simulink model "chotu_undir_2D"  (R2020a)
settings: Solver=VariableStepAuto  StartTime=0.0  StopTime=30  RelTol=1e-3
values from neighbouring files (symbols this model uses):
  J = 0.0001    [chotu_undir_parameters.m]
  Kb = 0.190    (= 0.19)    [chotu_undir_parameters.m]
  Kf = 0.000025    (= 2.5e-05)    [chotu_undir_parameters.m]
  Km = 0.084    [chotu_undir_parameters.m]
  L = 0.5    [chotu_undir_parameters.m]
  R = 16    [chotu_undir_parameters.m]
undefined symbols (not defined in the file or in its folder): motorIP, motorSP
libraries: mobileRoboticsLib x3, mobileRoboticsTrainingLib x1, robotalgslib x1
settings Model: Creator=RAJENDRA PHUTANE  LastModifiedBy=RAJENDRA PHUTANE

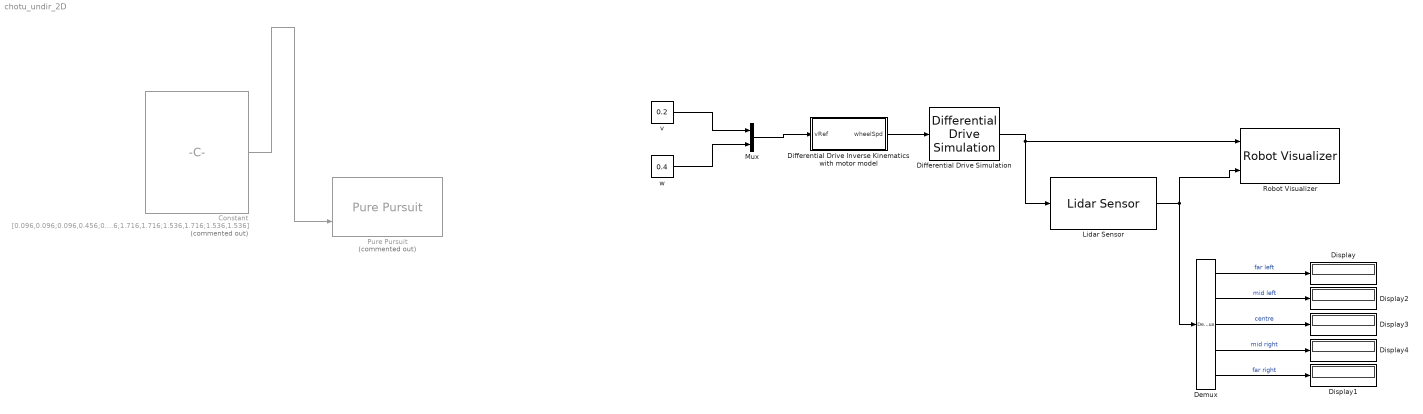
== system chotu_undir_2D ==
  Constant : Constant  Commented=on  Value=[0.096,0.096;0.096,0.456;0.278,0.456;0.278,0.096;1.356,0.096;1.356,0.186;0.996,0.544;0.996,0.740;1.086,0.816;1.6,0.276;2.616,0.276;2.616,0.456;1.716,0.456;1.716,0.636;1.896,0.636;1.896,1.176;1.716,1.176;1.716,1.356;1.896,1.356;1.896,1.536;1.716,1.536;1.716,1.716;1.536,1.716;1.536,1.536]
  Demux : Demux  Outputs=5
  Differential Drive Inverse Kinematics with motor model : Subsystem
  Differential Drive Simulation : mobileRoboticsLib/Kinematic Models/Differential Drive/Differential Drive Simulation  wheelRadius=wheelR  wheelBase=axleLength  initX=0.096  initY=0.096  initAngle=pi/2  Ts=0.1
      settings: SourceProductName=Mobile Robotics Simulation Toolbox
  Display{,1..4} (5 alike) : Display
  Lidar Sensor : mobileRoboticsLib/Environments/Lidar Sensor  mapName=map  sensorOffset=[0.04,0]  scanAngles=[-pi/2, -pi/4, 0, pi/4 , pi/2 ]  maxRange=5
      settings: SourceProductName=Mobile Robotics Simulation Toolbox
  Mux : Mux  Inputs=2
  Pure Pursuit : robotalgslib/Pure Pursuit  Commented=on  DesiredLinearVelocity=0.3  MaxAngularVelocity=inf  LookaheadDistance=0.15  TargetDirPort=off  SimulateUsing=Code generation
  Robot Visualizer : mobileRoboticsLib/Environments/Robot Visualizer  robotRadius=0.04  mapName=map  showTrajectory=on  hasWaypoints=off  hasLidar=on  sensorOffset=[0.04,0]  scanAngles=[-pi/2, -pi/4, 0, pi/4 , pi/2 ]  hasObjDetector=off  objDetectorOffset=[ 0, 0 ]  objDetectorAngle=0  objDetectorFOV=pi/4  objDetectorMaxRange=5  objectColors=[ 1, 0, 0; 0, 1, 0; 0, 0, 1 ]  objectMarkers=s
  v : Constant  Value=0.2  OutDataTypeStr=Inherit: Inherit via back propagation
  w : Constant  Value=0.4  OutDataTypeStr=Inherit: Inherit via back propagation
  wires:
  Demux/3 -> Display3/1  "centre"
  Demux/5 -> Display1/1  "far right"
  Demux/4 -> Display4/1  "mid right"
  Demux/2 -> Display2/1  "mid left"
  Differential Drive Inverse Kinematics with motor model/1(wheelSpd) -> Differential Drive Simulation/1
  Differential Drive Simulation/1 -> Lidar Sensor/1, Robot Visualizer/1
  Lidar Sensor/1 -> Robot Visualizer/2, Demux/1
  Demux/1 -> Display/1  "far left"
  Mux/1 -> Differential Drive Inverse Kinematics with motor model/1(vRef)
  Constant/1 -> Pure Pursuit/2
  v/1 -> Mux/1
  w/1 -> Mux/2

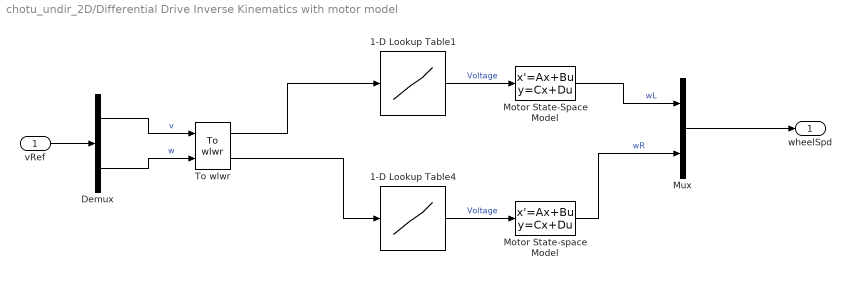
== system chotu_undir_2D/Differential Drive Inverse Kinematics with motor model ==
  vRef : Inport
  1-D Lookup Table1 : Lookup_n-D  NumberOfTableDimensions=1  BreakpointsForDimension1=motorSP  Table=motorIP  ExtrapMethod=Clip  InternalRulePriority=Speed  RndMeth=Simplest  InputSameDT=on
  1-D Lookup Table4 : Lookup_n-D  NumberOfTableDimensions=1  BreakpointsForDimension1=motorSP  Table=motorIP  ExtrapMethod=Clip  InternalRulePriority=Speed  RndMeth=Simplest  InputSameDT=on
  Demux : Demux  Outputs=2
  Motor State-Space Model : StateSpace  A=[-Kf/J Km/J; -Kb/L -R/L]  B=[0; 1/L]  C=[1 0]  D=[0]  InitialCondition=0
  Motor State-space Model : StateSpace  A=[-Kf/J Km/J; -Kb/L -R/L]  B=[0; 1/L]  C=[1 0]  D=[0]  InitialCondition=0
  Mux : Mux  Inputs=2
  To wlwr : mobileRoboticsTrainingLib/To wlwr  axleLength=axleLength  wheelR=wheelR
  wheelSpd : Outport  VectorParamsAs1DForOutWhenUnconnected=off
  wires:
  Demux/1 -> To wlwr/1  "v"
  vRef/1 -> Demux/1
  Demux/2 -> To wlwr/2  "w"
  Motor State-space Model/1 -> Mux/2  "wR"
  Mux/1 -> wheelSpd/1
  Motor State-Space Model/1 -> Mux/1  "wL"
  1-D Lookup Table4/1 -> Motor State-space Model/1  "Voltage"
  To wlwr/1 -> 1-D Lookup Table1/1
  To wlwr/2 -> 1-D Lookup Table4/1
  1-D Lookup Table1/1 -> Motor State-Space Model/1  "Voltage"
